simulink model "Passive"  (R2019a)
settings: Solver=VariableStepAuto  StartTime=0.0  StopTime=20.0  RelTol=1e-3
values from neighbouring files (symbols this model uses):
  b1 = 600    [code.m]
  b2 = 800    [code.m]
  k1 = 18000    [code.m]
  k2 = 1950000    [code.m]
  m1 = 350    [code.m]
  m2 = 40    [code.m]
settings Model: Creator=DEVASHISH  LastModifiedBy=DEVASHISH

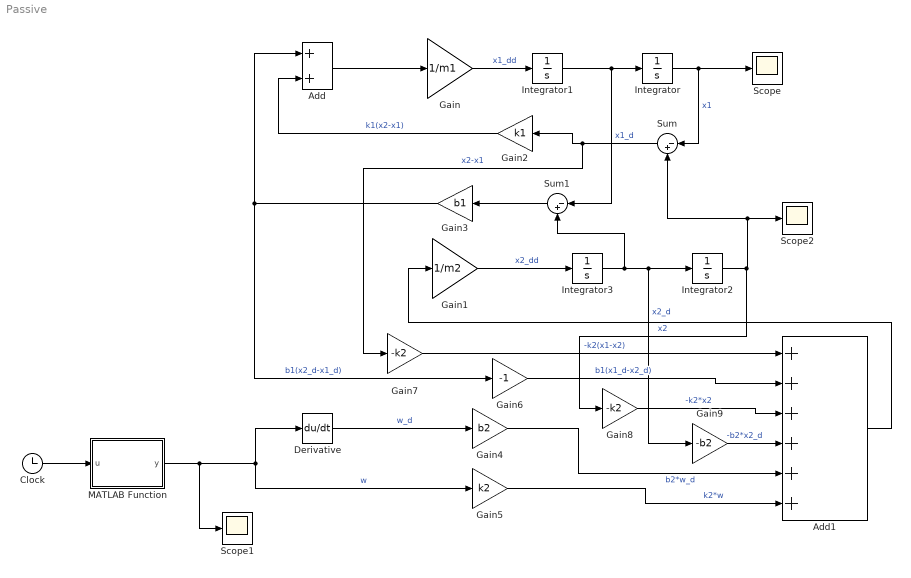
== system Passive ==
  Add : Sum
  Add1 : Sum  Inputs=++++++
  Clock : Clock
  Derivative : Derivative
  Gain : Gain  Gain=1/m1
  Gain1 : Gain  Gain=1/m2
  Gain2 : Gain  Gain=k1
  Gain3 : Gain  Gain=b1
  Gain4 : Gain  Gain=b2
  Gain5 : Gain  Gain=k2
  Gain6 : Gain  Gain=-1
  Gain7 : Gain  Gain=-k2
  Gain8 : Gain  Gain=-k2
  Gain9 : Gain  Gain=-b2
  Integrator{,1..3} (4 alike) : Integrator
  MATLAB Function : MATLAB Function  TreatAsAtomicUnit=on
  Scope : Scope
  Scope1 : Scope
  Scope2 : Scope
  Sum : Sum  Inputs=|-+
  Sum1 : Sum  Inputs=|-+
  wires:
  Integrator/1 -> Sum/1, Scope/1  "x1"
  Integrator1/1 -> Sum1/1, Integrator/1  "x1_d"
  Gain/1 -> Integrator1/1  "x1_dd"
  Integrator3/1 -> Sum1/2, Gain9/1, Integrator2/1  "x2_d"
  Integrator2/1 -> Sum/2, Scope2/1, Gain8/1  "x2"
  Gain1/1 -> Integrator3/1  "x2_dd"
  Sum/1 -> Gain7/1, Gain2/1  "x2-x1"
  Gain2/1 -> Add/2  "k1(x2-x1)"
  Sum1/1 -> Gain3/1
  Gain3/1 -> Add/1, Gain6/1  "b1(x2_d-x1_d)"
  Add/1 -> Gain/1
  MATLAB Function/1(y) -> Scope1/1, Derivative/1, Gain5/1  "w"
  Derivative/1 -> Gain4/1  "w_d"
  Gain5/1 -> Add1/6  "k2*w"
  Gain8/1 -> Add1/3  "-k2*x2"
  Gain9/1 -> Add1/4  "-b2*x2_d"
  Gain4/1 -> Add1/5  "b2*w_d"
  Gain6/1 -> Add1/2  "b1(x1_d-x2_d)"
  Gain7/1 -> Add1/1  "-k2(x1-x2)"
  Add1/1 -> Gain1/1
  Clock/1 -> MATLAB Function/1(u)

== matlab function Passive/MATLAB Function ==
  data: u input; y output
function y = fcn(u)
%if u>2
%y=1;
%if   u>5 && u<10
%y=-0.1*(5*(u-5)-(u-10))*sin(0.2*pi*u);
if u<8
    y=sin(0.25*pi*u);
else
y=0;
end
end
